simulink model "spherical_tank"  (R2017b)
settings: Solver=VariableStepAuto  StartTime=0.0  StopTime=200  RelTol=1e-3
values from neighbouring files (symbols this model uses):
  A = -1/((2*R*(sqrt(h0)))*(pi*(((a-b)^2)*(h0^2))/(H^2)+((2*b*(a-b))/H)*h0+b^2))    [init_canonical.m]    (also in init_spherical.m = (2*pi*(Rr-h0))/(pi*(2*Rr-h0)*h0)^2*(sqrt(h0)/(R)-Fu0)-1/(2*R)
  B = 1/(pi*(((a-b)^2)*(h0^2))/(H^2)+((2*b*(a-b))/H)*h0+b^2)    (= 3.04980111709)    [init_canonical.m]    (also in init_spherical.m = 1.97103532603)
  C = 1    [init_canonical.m]    (also in init_spherical.m)
  D = 0    [init_canonical.m]    (also in init_spherical.m)
  h0 = Fu0^2*R^2    (= 0.81)    [init_canonical.m]    (also in init_spherical.m = 0.2025)
  R = 900    [init_canonical.m]    (also in init_spherical.m = 30)
  Rr = 0.5    [init_spherical.m]
settings Model: Creator=Laci  LastModifiedBy=Laci

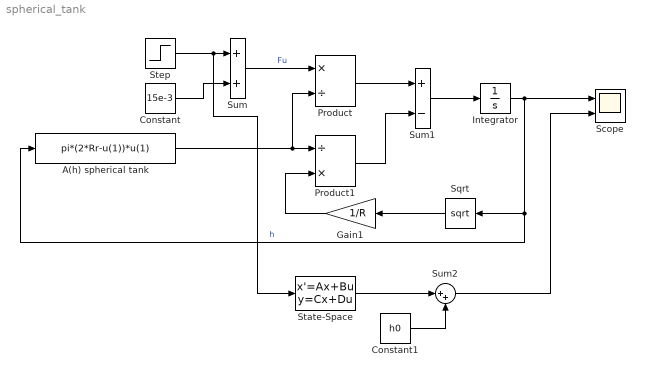
== system spherical_tank ==
  A(h) spherical tank : Fcn  Expr=pi*(2*Rr-u(1))*u(1)
  Constant : Constant  Value=15e-3
  Constant1 : Constant  Value=h0
  Gain1 : Gain  Gain=1/R
  Integrator : Integrator  InitialCondition=1e-3
  Product : Product  Inputs=*/
  Product1 : Product  Inputs=/*
  Scope : Scope  NumInputPorts=2
  Sqrt : Sqrt  SaturateOnIntegerOverflow=on
  State-Space : StateSpace  A=A  B=B  C=C  D=D  InitialCondition=0
  Step : Step  Time=100  After=1e-3  SampleTime=0
  Sum : Sum
  Sum1 : Sum  Inputs=+-
  Sum2 : Sum  Inputs=|++
  wires:
  Step/1 -> State-Space/1, Sum/1
  Constant/1 -> Sum/2
  Sum/1 -> Product/1  "Fu"
  Product/1 -> Sum1/1
  Sum1/1 -> Integrator/1
  Integrator/1 -> Scope/1, A(h) spherical tank/1, Sqrt/1  "h"
  Product1/1 -> Sum1/2
  State-Space/1 -> Sum2/1
  Constant1/1 -> Sum2/2
  Sum2/1 -> Scope/2
  Sqrt/1 -> Gain1/1
  A(h) spherical tank/1 -> Product/2, Product1/1
  Gain1/1 -> Product1/2
